simulink model "FieldOrientedControl"  (R2022b)
settings: configuration reference "FieldOrientedControl_ConfigSet" (kept outside this file)
PreLoadFcn:
  | run_start;
undefined symbols (not defined in the file or in its folder): DiscIntNeverNeededParam, dq_decouping_ena, dq_voltage_ratio, duty_sat_lower, duty_sat_upper, I_s_max, KI_c, Kp_c, L_d, L_q, p, Psi_p, svpwm_ena, task_time_mtrctrl
libraries: simulink x4
settings Model: DataDictionary=FieldOrientedControl.sldd  Creator=ext-turaim  LastModifiedBy=Musaab
settings ConfigSetRef: SourceName=FieldOrientedControl_ConfigSet

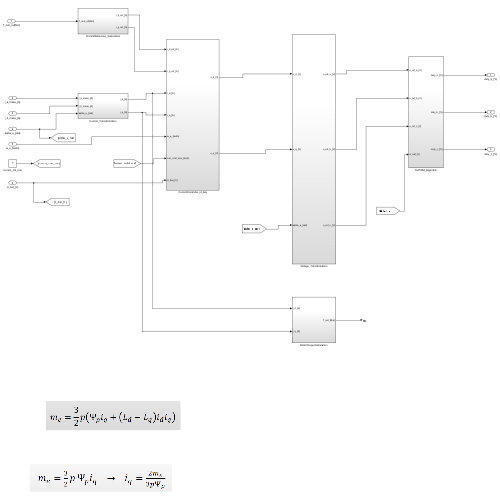
[thumbnail: Simulink's stored preview of the top-level diagram]
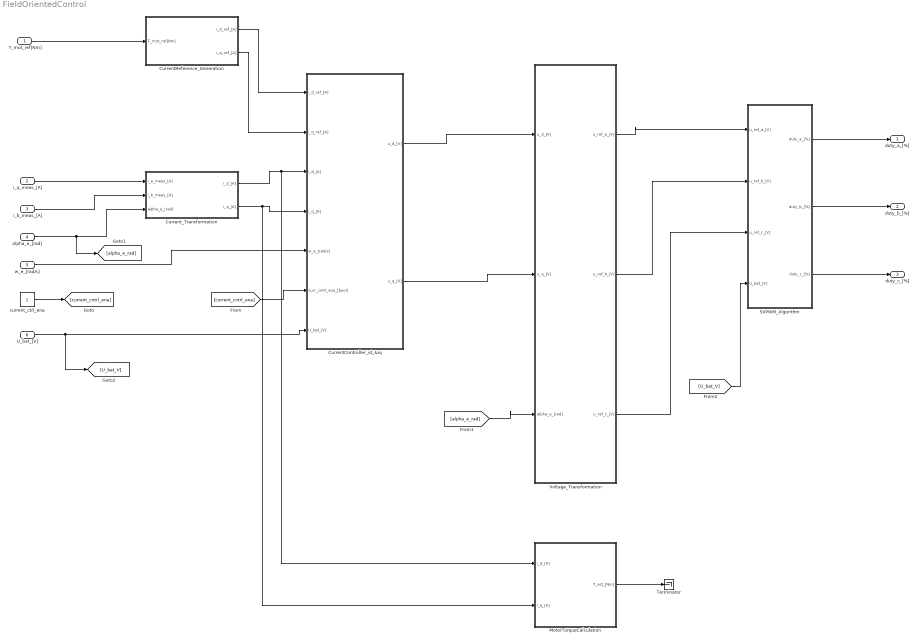
== system FieldOrientedControl ==
  T_mot_ref[Nm] : Inport  OutDataTypeStr=single  SampleTime=task_time_mtrctrl
  i_a_meas_[A] : Inport  Port=2  SampleTime=task_time_mtrctrl
  i_b_meas_[A] : Inport  Port=3  SampleTime=task_time_mtrctrl
  alpha_e_[rad] : Inport  Port=4  OutDataTypeStr=single  SampleTime=task_time_mtrctrl
  w_e_[rad/s] : Inport  Port=5  OutDataTypeStr=single  SampleTime=task_time_mtrctrl
  U_bat_[V] : Inport  Port=6  OutDataTypeStr=single  SampleTime=task_time_mtrctrl
  CurrentController_id_&iq : Subsystem
  CurrentReference_Generation : Subsystem
  Current_Transformation : Subsystem
  MotorTorqueCalculation : Subsystem
  SVPWM_Algorithm : Subsystem
  Terminator : Terminator
  Voltage_Transformation : Subsystem
  current_ctrl_ena : Constant  OutDataTypeStr=boolean  SampleTime=task_time_mtrctrl
  duty_a_[%] : Outport
  duty_b_[%] : Outport  Port=2
  duty_c_[%] : Outport  Port=3
  wires:
  i_a_meas_[A]/1 -> Current_Transformation/1(i_a_meas_[A])
  i_b_meas_[A]/1 -> Current_Transformation/2(i_b_meas_[A])
  alpha_e_[rad]/1 -> [alpha_e_rad], Current_Transformation/3(alpha_e_[rad])
  T_mot_ref[Nm]/1 -> CurrentReference_Generation/1(T_mot_ref[Nm])
  CurrentReference_Generation/1(i_d_ref_[A]) -> CurrentController_id_&iq/1(i_d_ref_[A])
  CurrentReference_Generation/2(i_q_ref_[A]) -> CurrentController_id_&iq/2(i_q_ref_[A])
  Current_Transformation/1(i_d_[A]) -> MotorTorqueCalculation/1(i_d_[A]), CurrentController_id_&iq/3(i_d_[A])
  Current_Transformation/2(i_q_[A]) -> MotorTorqueCalculation/2(i_q_[A]), CurrentController_id_&iq/4(i_q_[A])
  current_ctrl_ena/1 -> [current_cntrl_ena]
  [current_cntrl_ena] -> CurrentController_id_&iq/6(curr_cntrl_ena_[bool])
  w_e_[rad/s]/1 -> CurrentController_id_&iq/5(w_e_[rad/s])
  U_bat_[V]/1 -> [U_bat_V], CurrentController_id_&iq/7(U_bat_[V])
  CurrentController_id_&iq/1(u_d_[V]) -> Voltage_Transformation/1(u_d_[V])
  CurrentController_id_&iq/2(u_q_[V]) -> Voltage_Transformation/2(u_q_[V])
  [alpha_e_rad] -> Voltage_Transformation/3(alpha_e_[rad])
  Voltage_Transformation/1(u_ref_a_[V]) -> SVPWM_Algorithm/1(u_ref_a_[V])
  Voltage_Transformation/2(u_ref_b_[V]) -> SVPWM_Algorithm/2(u_ref_b_[V])
  Voltage_Transformation/3(u_ref_c_[V]) -> SVPWM_Algorithm/3(u_ref_c_[V])
  [U_bat_V] -> SVPWM_Algorithm/4(U_bat_[V])
  SVPWM_Algorithm/1(duty_a_[%]) -> duty_a_[%]/1
  SVPWM_Algorithm/2(duty_b_[%]) -> duty_b_[%]/1
  SVPWM_Algorithm/3(duty_c_[%]) -> duty_c_[%]/1
  MotorTorqueCalculation/1(T_act_[Nm]) -> Terminator/1

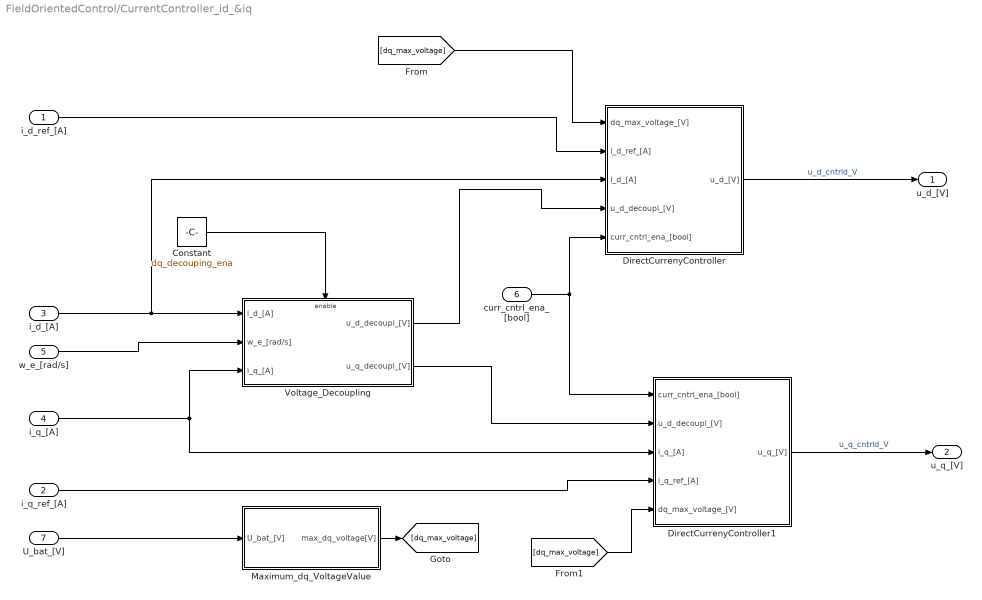
== system FieldOrientedControl/CurrentController_id_&iq ==
  i_d_ref_[A] : Inport
  i_q_ref_[A] : Inport  Port=2
  i_d_[A] : Inport  Port=3
  i_q_[A] : Inport  Port=4
  w_e_[rad/s] : Inport  Port=5
  curr_cntrl_ena_[bool] : Inport  Port=6
  U_bat_[V] : Inport  Port=7
  Constant : Constant  Value=dq_decouping_ena
  DirectCurrenyController : Subsystem
  DirectCurrenyController1 : Subsystem
  Maximum_dq_VoltageValue : Subsystem
  Voltage_Decoupling : Subsystem
  u_d_[V] : Outport
  u_q_[V] : Outport  Port=2
  wires:
  w_e_[rad/s]/1 -> Voltage_Decoupling/2(w_e_[rad/s])
  i_d_[A]/1 -> Voltage_Decoupling/1(i_d_[A]), DirectCurrenyController/3(i_d_[A])
  i_q_[A]/1 -> Voltage_Decoupling/3(i_q_[A]), DirectCurrenyController1/3(i_q_[A])
  i_d_ref_[A]/1 -> DirectCurrenyController/2(i_d_ref_[A])
  Voltage_Decoupling/1(u_d_decoupl_[V]) -> DirectCurrenyController/4(u_d_decoupl_[V])
  curr_cntrl_ena_[bool]/1 -> DirectCurrenyController1/1(curr_cntrl_ena_[bool]), DirectCurrenyController/5(curr_cntrl_ena_[bool])
  U_bat_[V]/1 -> Maximum_dq_VoltageValue/1(U_bat_[V])
  Maximum_dq_VoltageValue/1(max_dq_voltage[V]) -> [dq_max_voltage]
  [dq_max_voltage] -> DirectCurrenyController/1(dq_max_voltage_[V])
  DirectCurrenyController/1(u_d_[V]) -> u_d_[V]/1  "u_d_cntrld_V"
  [dq_max_voltage] -> DirectCurrenyController1/5(dq_max_voltage_[V])
  Voltage_Decoupling/2(u_q_decoupl_[V]) -> DirectCurrenyController1/2(u_d_decoupl_[V])
  i_q_ref_[A]/1 -> DirectCurrenyController1/4(i_q_ref_[A])
  DirectCurrenyController1/1(u_q_[V]) -> u_q_[V]/1  "u_q_cntrld_V"
  Constant/1 -> Voltage_Decoupling/Enable

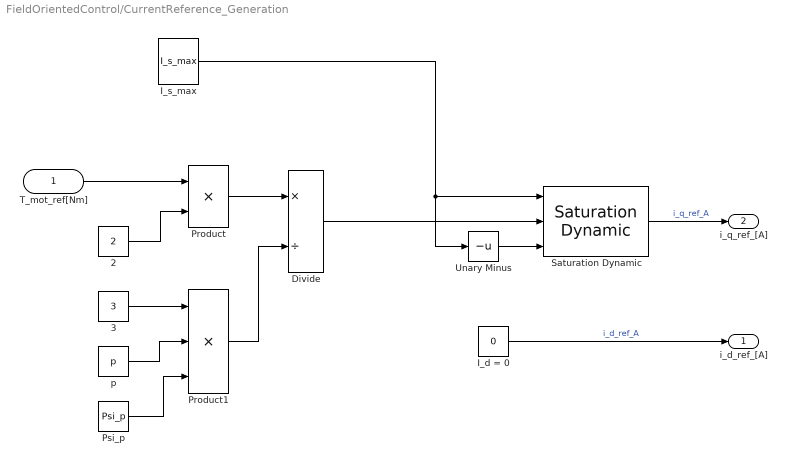
== system FieldOrientedControl/CurrentReference_Generation ==
  T_mot_ref[Nm] : Inport
  2 : Constant  Value=2  OutDataTypeStr=single
  3 : Constant  Value=3  OutDataTypeStr=single
  Divide : Product  Inputs=*/
  I_d = 0 : Constant  Value=0  OutDataTypeStr=single
  I_s_max : Constant  Value=I_s_max
  Product : Product
  Product1 : Product  Inputs=3
  Psi_p : Constant  Value=Psi_p  OutDataTypeStr=single
  Saturation Dynamic : simulink/Discontinuities/Saturation Dynamic  OutMin=[]  OutMax=[]  OutDataTypeStr=Inherit: Same as second input  OutDataType=fixdt(1, 16)  OutScaling=2^-10  DoSatur=off
  Unary Minus : UnaryMinus
  p : Constant  Value=p  OutDataTypeStr=single
  i_d_ref_[A] : Outport
  i_q_ref_[A] : Outport  Port=2
  wires:
  T_mot_ref[Nm]/1 -> Product/1
  2/1 -> Product/2
  3/1 -> Product1/1
  p/1 -> Product1/2
  Psi_p/1 -> Product1/3
  Product/1 -> Divide/1
  Product1/1 -> Divide/2
  I_s_max/1 -> Unary Minus/1, Saturation Dynamic/1
  Divide/1 -> Saturation Dynamic/2
  Saturation Dynamic/1 -> i_q_ref_[A]/1  "i_q_ref_A"
  Unary Minus/1 -> Saturation Dynamic/3
  I_d = 0/1 -> i_d_ref_[A]/1  "i_d_ref_A"

== system FieldOrientedControl/Current_Transformation ==
  i_a_meas_[A] : Inport
  i_b_meas_[A] : Inport  Port=2
  alpha_e_[rad] : Inport  Port=3
  Clark_Transformation : Subsystem
  Park_Transformation : Subsystem
  i_d_[A] : Outport
  i_q_[A] : Outport  Port=2
  wires:
  i_a_meas_[A]/1 -> Clark_Transformation/1(i_a_meas_[A])
  i_b_meas_[A]/1 -> Clark_Transformation/2(i_b_meas_[A])
  Clark_Transformation/1(i_x_[A]) -> Park_Transformation/1(i_x_[A])  "i_x_meas_A"
  Clark_Transformation/2(i_y_[A]) -> Park_Transformation/2(i_y_[A])  "i_y_meas_A"
  alpha_e_[rad]/1 -> Park_Transformation/3(alpha_e_[rad])
  Park_Transformation/1(i_d_[A]) -> i_d_[A]/1  "i_d_meas_A"
  Park_Transformation/2(i_q_[A]) -> i_q_[A]/1  "i_q_meas_A"

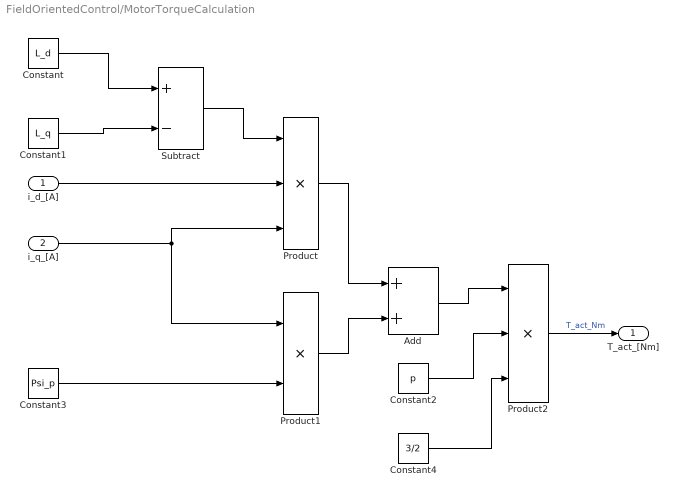
== system FieldOrientedControl/MotorTorqueCalculation ==
  i_d_[A] : Inport
  i_q_[A] : Inport  Port=2
  Add : Sum
  Constant : Constant  Value=L_d
  Constant1 : Constant  Value=L_q
  Constant2 : Constant  Value=p
  Constant3 : Constant  Value=Psi_p
  Constant4 : Constant  Value=3/2
  Product : Product  Inputs=3
  Product1 : Product
  Product2 : Product  Inputs=3
  Subtract : Sum  Inputs=+-
  T_act_[Nm] : Outport
  wires:
  Constant/1 -> Subtract/1
  Constant1/1 -> Subtract/2
  Subtract/1 -> Product/1
  i_d_[A]/1 -> Product/2
  i_q_[A]/1 -> Product1/1, Product/3
  Constant3/1 -> Product1/2
  Product/1 -> Add/1
  Product1/1 -> Add/2
  Add/1 -> Product2/1
  Constant2/1 -> Product2/2
  Constant4/1 -> Product2/3
  Product2/1 -> T_act_[Nm]/1  "T_act_Nm"

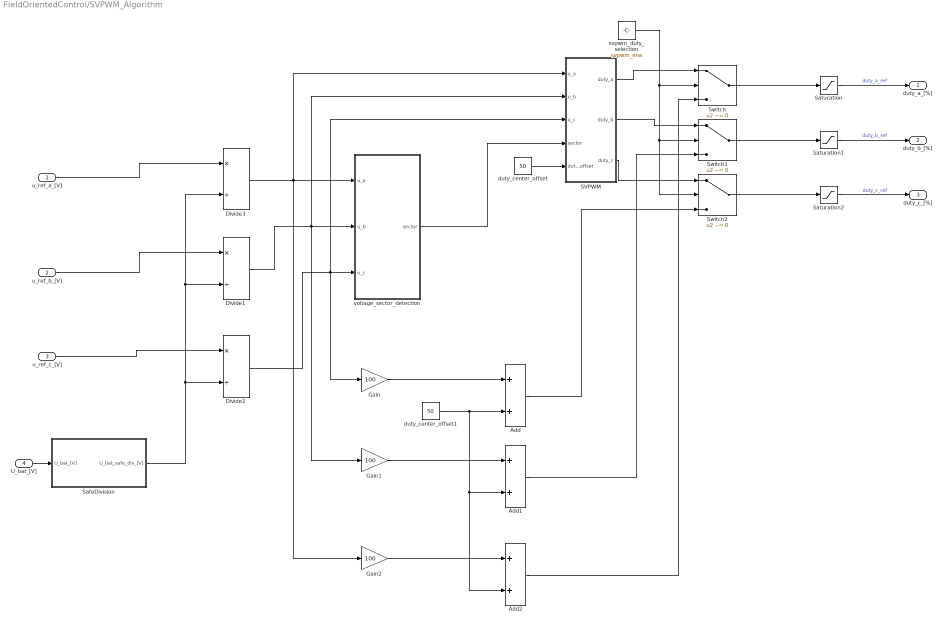
== system FieldOrientedControl/SVPWM_Algorithm ==
  u_ref_a_[V] : Inport
  u_ref_b_[V] : Inport  Port=2
  u_ref_c_[V] : Inport  Port=3
  U_bat_[V] : Inport  Port=4
  Add : Sum
  Add1 : Sum
  Add2 : Sum
  Divide1 : Product  Inputs=*/
  Divide2 : Product  Inputs=*/
  Divide3 : Product  Inputs=*/
  Gain : Gain  Gain=100
  Gain1 : Gain  Gain=100
  Gain2 : Gain  Gain=100
  SVPWM : Stateflow chart  TreatAsAtomicUnit=on
  SafeDivision : Subsystem
  Saturation : Saturate  UpperLimit=duty_sat_upper  LowerLimit=duty_sat_lower
  Saturation1 : Saturate  UpperLimit=duty_sat_upper  LowerLimit=duty_sat_lower
  Saturation2 : Saturate  UpperLimit=duty_sat_upper  LowerLimit=duty_sat_lower
  Switch : Switch  Criteria=u2 ~= 0  SaturateOnIntegerOverflow=off  InputSameDT=off
  Switch1 : Switch  Criteria=u2 ~= 0  SaturateOnIntegerOverflow=off  InputSameDT=off
  Switch2 : Switch  Criteria=u2 ~= 0  SaturateOnIntegerOverflow=off  InputSameDT=off
  duty_center_offset : Constant  Value=50  OutDataTypeStr=single
  duty_center_offset1 : Constant  Value=50  OutDataTypeStr=single
  svpwm_duty_selection : Constant  Value=svpwm_ena  OutDataTypeStr=single
  voltage_sector_detection : Stateflow chart  TreatAsAtomicUnit=on
  duty_a_[%] : Outport  OutDataTypeStr=single
  duty_b_[%] : Outport  Port=2  OutDataTypeStr=single
  duty_c_[%] : Outport  Port=3  OutDataTypeStr=single
  wires:
  U_bat_[V]/1 -> SafeDivision/1(U_bat_[V])
  u_ref_a_[V]/1 -> Divide3/1
  u_ref_b_[V]/1 -> Divide1/1
  u_ref_c_[V]/1 -> Divide2/1
  SafeDivision/1(U_bat_safe_div_[V]) -> Divide2/2, Divide1/2, Divide3/2
  Divide3/1 -> Gain2/1, voltage_sector_detection/1(u_a), SVPWM/1(u_a)
  Divide1/1 -> Gain1/1, voltage_sector_detection/2(u_b), SVPWM/2(u_b)
  Divide2/1 -> Gain/1, voltage_sector_detection/3(u_c), SVPWM/3(u_c)
  voltage_sector_detection/1(sector) -> SVPWM/4(sector)
  duty_center_offset/1 -> SVPWM/5(duty_offset)
  Gain/1 -> Add/1
  duty_center_offset1/1 -> Add2/2, Add1/2, Add/2
  Gain1/1 -> Add1/1
  Gain2/1 -> Add2/1
  SVPWM/1(duty_a) -> Switch/1
  SVPWM/2(duty_b) -> Switch1/1
  SVPWM/3(duty_c) -> Switch2/1
  Add2/1 -> Switch/3
  Add1/1 -> Switch1/3
  Add/1 -> Switch2/3
  svpwm_duty_selection/1 -> Switch1/2, Switch2/2, Switch/2
  Switch/1 -> Saturation/1
  Switch2/1 -> Saturation2/1
  Switch1/1 -> Saturation1/1
  Saturation2/1 -> duty_c_[%]/1  "duty_c_ref"
  Saturation1/1 -> duty_b_[%]/1  "duty_b_ref"
  Saturation/1 -> duty_a_[%]/1  "duty_a_ref"

== system FieldOrientedControl/Voltage_Transformation ==
  u_d_[V] : Inport
  u_q_[V] : Inport  Port=2
  alpha_e_[rad] : Inport  Port=3
  Inverse_Clarke_Transform : Subsystem
  Inverse_Park_Transform : Subsystem
  u_ref_a_[V] : Outport
  u_ref_b_[V] : Outport  Port=2
  u_ref_c_[V] : Outport  Port=3
  wires:
  u_d_[V]/1 -> Inverse_Park_Transform/1(u_d_[V])
  u_q_[V]/1 -> Inverse_Park_Transform/2(u_q_[V])
  alpha_e_[rad]/1 -> Inverse_Park_Transform/3(alpha_e_[rad])
  Inverse_Park_Transform/1(u_x_[V]) -> Inverse_Clarke_Transform/1(u_x_[V])  "u_x_V"
  Inverse_Park_Transform/2(u_y_[V]) -> Inverse_Clarke_Transform/2(u_y_[V])  "u_y_V"
  Inverse_Clarke_Transform/1(u_ref_a_[V]) -> u_ref_a_[V]/1  "u_ref_a_V"
  Inverse_Clarke_Transform/2(u_ref_b_[V]) -> u_ref_b_[V]/1  "u_ref_b_V"
  Inverse_Clarke_Transform/3(u_ref_c_[V]) -> u_ref_c_[V]/1  "u_ref_c_V"

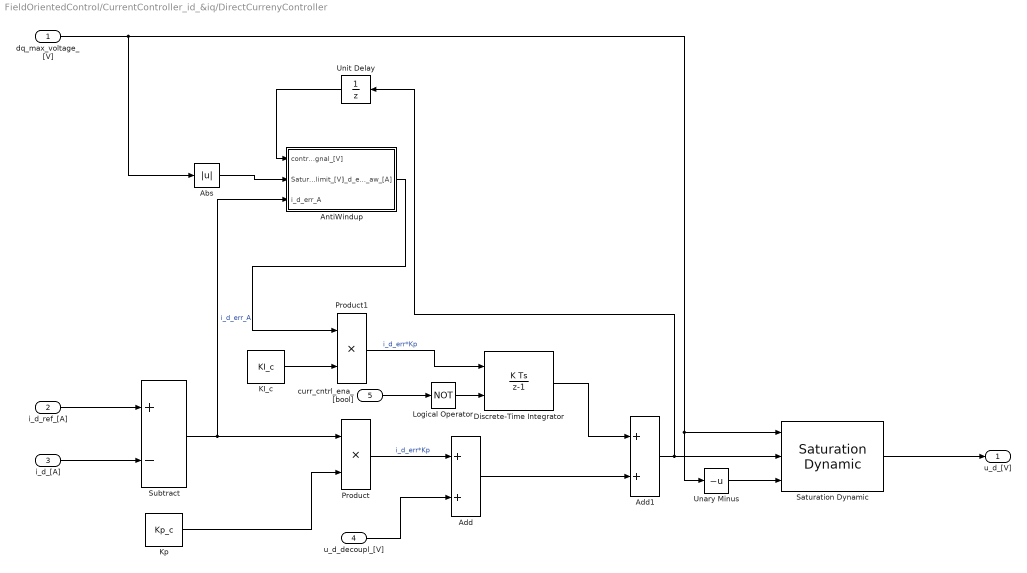
== system FieldOrientedControl/CurrentController_id_&iq/DirectCurrenyController ==
  dq_max_voltage_[V] : Inport
  i_d_ref_[A] : Inport  Port=2
  i_d_[A] : Inport  Port=3
  u_d_decoupl_[V] : Inport  Port=4
  curr_cntrl_ena_[bool] : Inport  Port=5
  Abs : Abs  SaturateOnIntegerOverflow=off
  Add : Sum
  Add1 : Sum
  AntiWindup : Subsystem
  Discrete-Time Integrator : DiscreteIntegrator  ExternalReset=level  SampleTime=-1  ICPrevOutput=DiscIntNeverNeededParam  ICPrevScaledInput=DiscIntNeverNeededParam
  KI_c : Constant  Value=KI_c
  Kp : Constant  Value=Kp_c
  Logical Operator : Logic  Operator=NOT  AllPortsSameDT=off  OutDataTypeStr=boolean
  Product : Product
  Product1 : Product
  Saturation Dynamic : simulink/Discontinuities/Saturation Dynamic  OutMin=[]  OutMax=[]  OutDataTypeStr=Inherit: Same as second input  OutDataType=fixdt(1, 16)  OutScaling=2^-10  DoSatur=off
  Subtract : Sum  Inputs=+-
  Unary Minus : UnaryMinus
  Unit Delay : UnitDelay  SampleTime=-1  HasFrameUpgradeWarning=on
  u_d_[V] : Outport
  wires:
  i_d_ref_[A]/1 -> Subtract/1
  i_d_[A]/1 -> Subtract/2
  Kp/1 -> Product/2
  Subtract/1 -> Product/1, AntiWindup/3(i_d_err_A)  "i_d_err_A"
  Product/1 -> Add/1  "i_d_err*Kp"
  u_d_decoupl_[V]/1 -> Add/2
  KI_c/1 -> Product1/2
  Product1/1 -> Discrete-Time Integrator/1  "i_d_err*Kp"
  Logical Operator/1 -> Discrete-Time Integrator/2
  curr_cntrl_ena_[bool]/1 -> Logical Operator/1
  Add/1 -> Add1/2
  Discrete-Time Integrator/1 -> Add1/1
  Add1/1 -> Unit Delay/1, Saturation Dynamic/2
  dq_max_voltage_[V]/1 -> Abs/1, Unary Minus/1, Saturation Dynamic/1
  Unary Minus/1 -> Saturation Dynamic/3
  Saturation Dynamic/1 -> u_d_[V]/1
  Unit Delay/1 -> AntiWindup/1(control_signal_[V])
  Abs/1 -> AntiWindup/2(Saturation_limit_[V])
  AntiWindup/1(i_d_err_aw_[A]) -> Product1/1

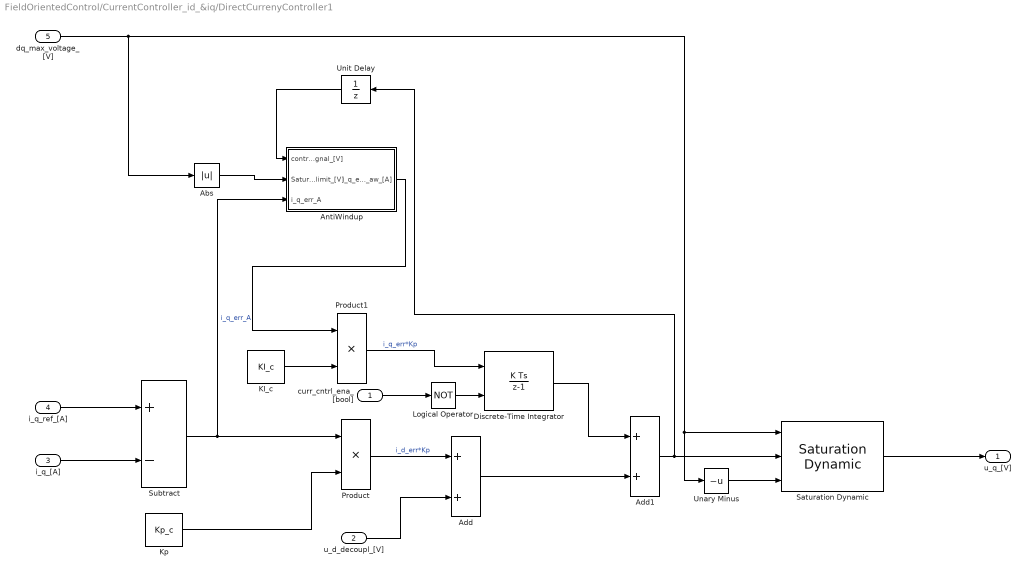
== system FieldOrientedControl/CurrentController_id_&iq/DirectCurrenyController1 ==
  curr_cntrl_ena_[bool] : Inport
  u_d_decoupl_[V] : Inport  Port=2
  i_q_[A] : Inport  Port=3
  i_q_ref_[A] : Inport  Port=4
  dq_max_voltage_[V] : Inport  Port=5
  Abs : Abs  SaturateOnIntegerOverflow=off
  Add : Sum
  Add1 : Sum
  AntiWindup : Subsystem
  Discrete-Time Integrator : DiscreteIntegrator  ExternalReset=level  SampleTime=-1  ICPrevOutput=DiscIntNeverNeededParam  ICPrevScaledInput=DiscIntNeverNeededParam
  KI_c : Constant  Value=KI_c
  Kp : Constant  Value=Kp_c
  Logical Operator : Logic  Operator=NOT  AllPortsSameDT=off  OutDataTypeStr=boolean
  Product : Product
  Product1 : Product
  Saturation Dynamic : simulink/Discontinuities/Saturation Dynamic  OutMin=[]  OutMax=[]  OutDataTypeStr=Inherit: Same as second input  OutDataType=fixdt(1, 16)  OutScaling=2^-10  DoSatur=off
  Subtract : Sum  Inputs=+-
  Unary Minus : UnaryMinus
  Unit Delay : UnitDelay  SampleTime=-1  HasFrameUpgradeWarning=on
  u_q_[V] : Outport
  wires:
  AntiWindup/1(i_q_err_aw_[A]) -> Product1/1
  Abs/1 -> AntiWindup/2(Saturation_limit_[V])
  Unit Delay/1 -> AntiWindup/1(control_signal_[V])
  Saturation Dynamic/1 -> u_q_[V]/1
  Unary Minus/1 -> Saturation Dynamic/3
  dq_max_voltage_[V]/1 -> Saturation Dynamic/1, Unary Minus/1, Abs/1
  Add1/1 -> Saturation Dynamic/2, Unit Delay/1
  Discrete-Time Integrator/1 -> Add1/1
  Add/1 -> Add1/2
  curr_cntrl_ena_[bool]/1 -> Logical Operator/1
  Logical Operator/1 -> Discrete-Time Integrator/2
  Product1/1 -> Discrete-Time Integrator/1  "i_q_err*Kp"
  KI_c/1 -> Product1/2
  u_d_decoupl_[V]/1 -> Add/2
  Product/1 -> Add/1  "i_d_err*Kp"
  Subtract/1 -> AntiWindup/3(i_q_err_A), Product/1  "i_q_err_A"
  Kp/1 -> Product/2
  i_q_[A]/1 -> Subtract/2
  i_q_ref_[A]/1 -> Subtract/1

== system FieldOrientedControl/CurrentController_id_&iq/Maximum_dq_VoltageValue ==
  U_bat_[V] : Inport
  1/sqrt(3) : Constant  Value=dq_voltage_ratio
  Product : Product
  max_dq_voltage[V] : Outport
  wires:
  U_bat_[V]/1 -> Product/1
  Product/1 -> max_dq_voltage[V]/1  "dq_max_voltage_V"
  1/sqrt(3)/1 -> Product/2

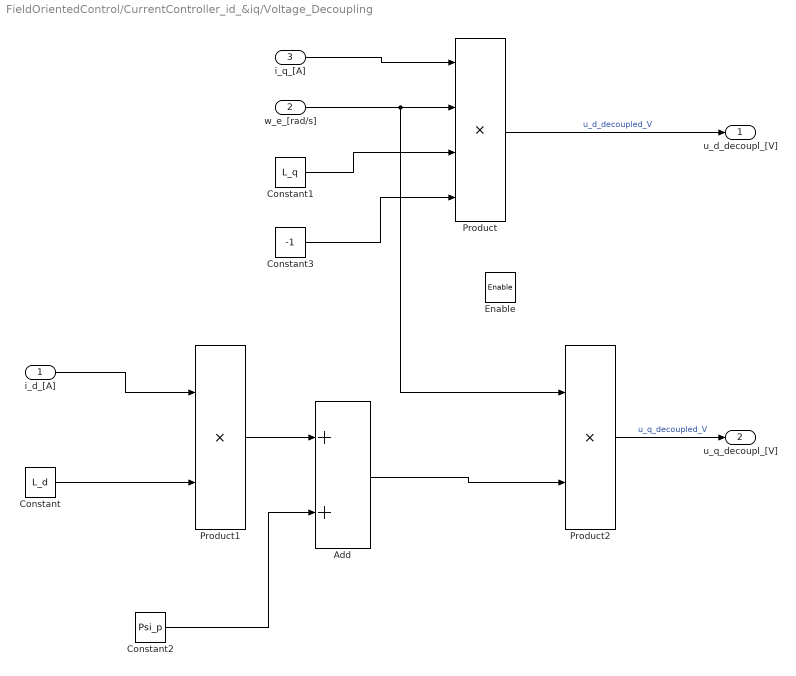
== system FieldOrientedControl/CurrentController_id_&iq/Voltage_Decoupling ==
  i_d_[A] : Inport
  w_e_[rad/s] : Inport  Port=2
  i_q_[A] : Inport  Port=3
  Enable : EnablePort
  Add : Sum
  Constant : Constant  Value=L_d
  Constant1 : Constant  Value=L_q
  Constant2 : Constant  Value=Psi_p
  Constant3 : Constant  Value=-1  OutDataTypeStr=single
  Product : Product  Inputs=4
  Product1 : Product
  Product2 : Product
  u_d_decoupl_[V] : Outport
  u_q_decoupl_[V] : Outport  Port=2
  wires:
  i_q_[A]/1 -> Product/1
  w_e_[rad/s]/1 -> Product2/1, Product/2
  Constant1/1 -> Product/3
  Constant3/1 -> Product/4
  Product/1 -> u_d_decoupl_[V]/1  "u_d_decoupled_V"
  i_d_[A]/1 -> Product1/1
  Constant/1 -> Product1/2
  Product1/1 -> Add/1
  Constant2/1 -> Add/2
  Add/1 -> Product2/2
  Product2/1 -> u_q_decoupl_[V]/1  "u_q_decoupled_V"

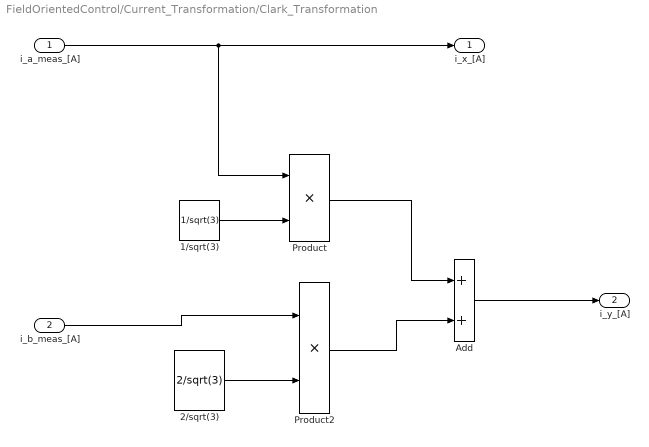
== system FieldOrientedControl/Current_Transformation/Clark_Transformation ==
  i_a_meas_[A] : Inport
  i_b_meas_[A] : Inport  Port=2
  1/sqrt(3) : Constant  Value=1/sqrt(3)  OutDataTypeStr=single
  2/sqrt(3) : Constant  Value=2/sqrt(3)  OutDataTypeStr=single
  Add : Sum
  Product : Product
  Product2 : Product
  i_x_[A] : Outport
  i_y_[A] : Outport  Port=2
  wires:
  i_a_meas_[A]/1 -> Product/1, i_x_[A]/1
  1/sqrt(3)/1 -> Product/2
  i_b_meas_[A]/1 -> Product2/1
  2/sqrt(3)/1 -> Product2/2
  Product/1 -> Add/1
  Product2/1 -> Add/2
  Add/1 -> i_y_[A]/1

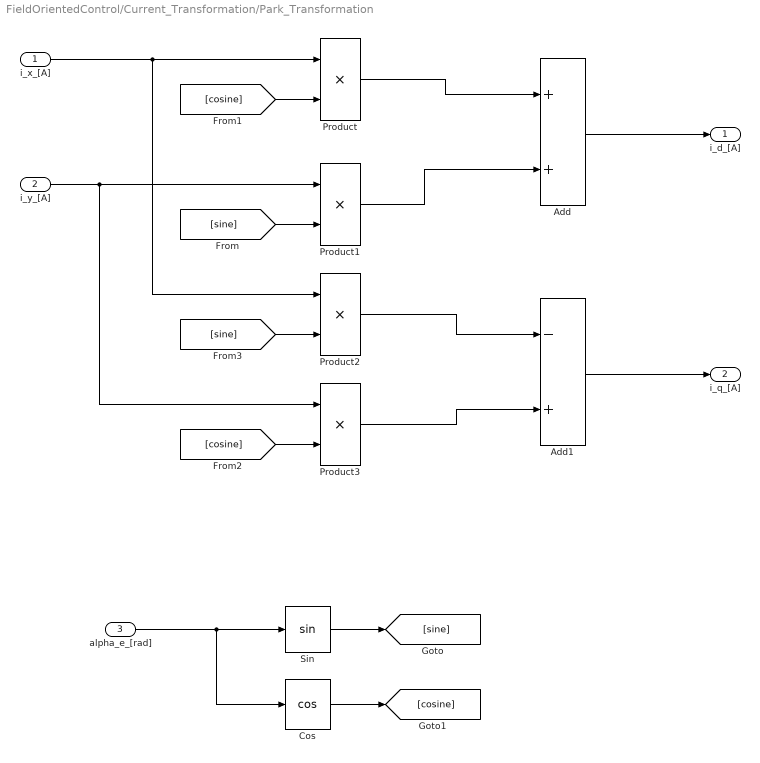
== system FieldOrientedControl/Current_Transformation/Park_Transformation ==
  i_x_[A] : Inport
  i_y_[A] : Inport  Port=2
  alpha_e_[rad] : Inport  Port=3
  Add : Sum
  Add1 : Sum  Inputs=-+
  Cos : Trigonometry  Operator=cos
  Product{,1..3} (4 alike) : Product
  Sin : Trigonometry
  i_d_[A] : Outport
  i_q_[A] : Outport  Port=2
  wires:
  alpha_e_[rad]/1 -> Cos/1, Sin/1
  Sin/1 -> [sine]
  Cos/1 -> [cosine]
  i_x_[A]/1 -> Product2/1, Product/1
  [cosine] -> Product/2
  i_y_[A]/1 -> Product3/1, Product1/1
  [cosine] -> Product3/2
  [sine] -> Product2/2
  [sine] -> Product1/2
  Product/1 -> Add/1
  Product1/1 -> Add/2
  Add/1 -> i_d_[A]/1
  Product2/1 -> Add1/1
  Product3/1 -> Add1/2
  Add1/1 -> i_q_[A]/1

== system FieldOrientedControl/SVPWM_Algorithm/SafeDivision ==
  U_bat_[V] : Inport
  Compare To Constant : simulink/Logic and Bit Operations/Compare To Constant  relop===  const=0  OutDataTypeStr=boolean
  Constant : Constant  Value=1e-6
  Switch : Switch  Criteria=u2 ~= 0  SaturateOnIntegerOverflow=off  InputSameDT=off
  U_bat_safe_div_[V] : Outport
  wires:
  Compare To Constant/1 -> Switch/2
  U_bat_[V]/1 -> Switch/3, Compare To Constant/1
  Constant/1 -> Switch/1
  Switch/1 -> U_bat_safe_div_[V]/1

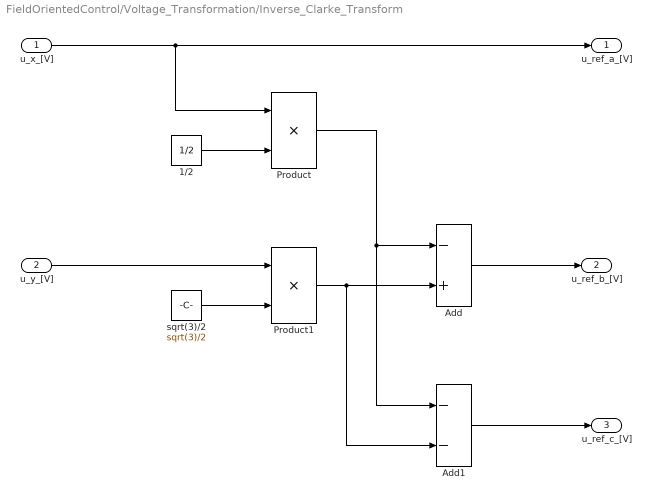
== system FieldOrientedControl/Voltage_Transformation/Inverse_Clarke_Transform ==
  u_x_[V] : Inport
  u_y_[V] : Inport  Port=2
  1/2 : Constant  Value=1/2  OutDataTypeStr=single
  Add : Sum  Inputs=-+
  Add1 : Sum  Inputs=--
  Product : Product
  Product1 : Product
  sqrt(3)/2 : Constant  Value=sqrt(3)/2  OutDataTypeStr=single
  u_ref_a_[V] : Outport
  u_ref_b_[V] : Outport  Port=2
  u_ref_c_[V] : Outport  Port=3
  wires:
  u_x_[V]/1 -> Product/1, u_ref_a_[V]/1
  1/2/1 -> Product/2
  sqrt(3)/2/1 -> Product1/2
  u_y_[V]/1 -> Product1/1
  Product1/1 -> Add1/2, Add/2
  Product/1 -> Add1/1, Add/1
  Add/1 -> u_ref_b_[V]/1
  Add1/1 -> u_ref_c_[V]/1

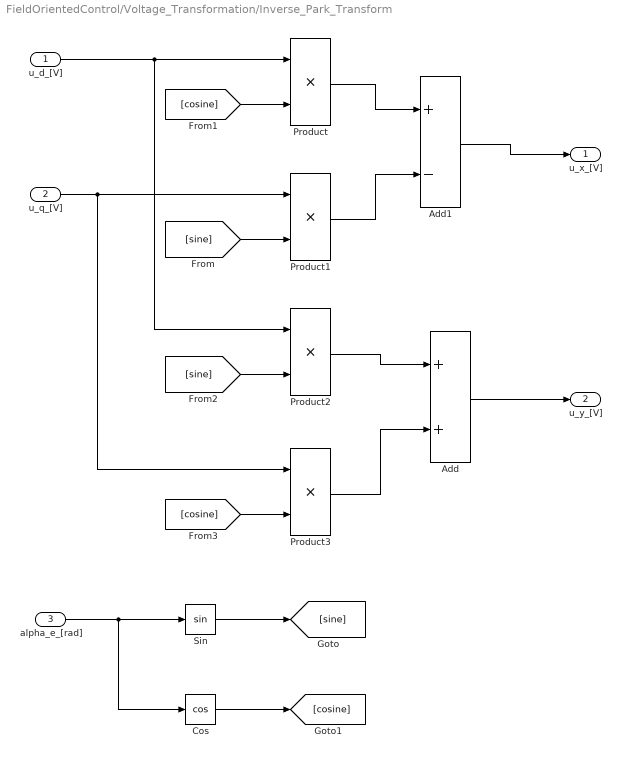
== system FieldOrientedControl/Voltage_Transformation/Inverse_Park_Transform ==
  u_d_[V] : Inport
  u_q_[V] : Inport  Port=2
  alpha_e_[rad] : Inport  Port=3
  Add : Sum
  Add1 : Sum  Inputs=+-
  Cos : Trigonometry  Operator=cos
  Product{,1..3} (4 alike) : Product
  Sin : Trigonometry
  u_x_[V] : Outport
  u_y_[V] : Outport  Port=2
  wires:
  alpha_e_[rad]/1 -> Cos/1, Sin/1
  Sin/1 -> [sine]
  Cos/1 -> [cosine]
  u_d_[V]/1 -> Product2/1, Product/1
  [sine] -> Product1/2
  [cosine] -> Product/2
  u_q_[V]/1 -> Product3/1, Product1/1
  [sine] -> Product2/2
  [cosine] -> Product3/2
  Product2/1 -> Add/1
  Product3/1 -> Add/2
  Add/1 -> u_y_[V]/1
  Product/1 -> Add1/1
  Product1/1 -> Add1/2
  Add1/1 -> u_x_[V]/1

== system FieldOrientedControl/CurrentController_id_&iq/DirectCurrenyController/AntiWindup ==
  control_signal_[V] : Inport
  Saturation_limit_[V] : Inport  Port=2
  i_d_err_A : Inport  Port=3
  Abs : Abs  SaturateOnIntegerOverflow=off
  Product : Product
  Relational Operator : RelationalOperator  Operator=<  OutDataTypeStr=boolean  RndMeth=Simplest  InputSameDT=off
  i_d_err_aw_[A] : Outport
  wires:
  control_signal_[V]/1 -> Abs/1
  Abs/1 -> Relational Operator/1
  Saturation_limit_[V]/1 -> Relational Operator/2
  Relational Operator/1 -> Product/1
  i_d_err_A/1 -> Product/2
  Product/1 -> i_d_err_aw_[A]/1

== system FieldOrientedControl/CurrentController_id_&iq/DirectCurrenyController1/AntiWindup ==
  control_signal_[V] : Inport
  Saturation_limit_[V] : Inport  Port=2
  i_q_err_A : Inport  Port=3
  Abs : Abs  SaturateOnIntegerOverflow=off
  Product : Product
  Relational Operator : RelationalOperator  Operator=<  OutDataTypeStr=boolean  RndMeth=Simplest  InputSameDT=off
  i_q_err_aw_[A] : Outport
  wires:
  Product/1 -> i_q_err_aw_[A]/1
  i_q_err_A/1 -> Product/2
  Relational Operator/1 -> Product/1
  Saturation_limit_[V]/1 -> Relational Operator/2
  Abs/1 -> Relational Operator/1
  control_signal_[V]/1 -> Abs/1

== stateflow chart FieldOrientedControl/SVPWM_Algorithm/SVPWM ==
  note: ?
  (default) -> (junction 15)
  (junction 15) -> (junction 17) [order 1] : [sector == 1 || sector == 4]{
      |
      | duty_a = duty_offset + duty_offset*(u_a - u_c);
      | duty_b = duty_offset + duty_offset*(2*u_b - u_a - u_c);
      | duty_c = duty_offset + duty_offset*(u_c - u_a);
      |
      | }
  (junction 15) -> (junction 19) [order 2]
  (junction 19) -> (junction 20) [order 1] : [sector == 2 || sector == 5]{
      |
      | duty_a = duty_offset + duty_offset*(2*u_a - u_b - u_c);
      | duty_b = duty_offset + duty_offset*(u_b - u_c);
      | duty_c = duty_offset + duty_offset*(u_c - u_b);
      |
      | }
  (junction 19) -> (junction 23) [order 2]
  (junction 23) -> (junction 24) : [sector == 3 || sector == 6]{
      |
      | duty_a = duty_offset + duty_offset*(u_a - u_b);
      | duty_b = duty_offset + duty_offset*(u_b - u_a);
      | duty_c = duty_offset + duty_offset*(2*u_c - u_a - u_b);
      |
      | }
  data: u_a input; u_b input; u_c input; sector input; duty_a output; duty_b output; duty_c output; duty_offset input

== stateflow chart FieldOrientedControl/SVPWM_Algorithm/voltage_sector_detection ==
  (default) -> (junction 4)
  (junction 4) -> (junction 20) [order 2]
  (junction 4) -> (junction 6) [order 1] : [u_a >= u_b]
  (junction 20) -> (junction 21)
  (junction 21) -> (junction 22) [order 1] : [u_a >= u_c]{sector = 2}
  (junction 6) -> (junction 7) [order 1] : [u_c >= u_a]{sector = 5}
  (junction 6) -> (junction 11) [order 2]
  (junction 21) -> (junction 26) [order 2]
  (junction 26) -> (junction 27) [order 1] : [u_b >= u_c]{sector = 3}
  (junction 26) -> (junction 31) [order 2]
  (junction 11) -> (junction 14) [order 1] : [u_c >= u_b]{sector = 6}
  (junction 11) -> (junction 16) [order 2]
  (junction 16) -> (junction 17) : {sector = 1}
  (junction 31) -> (junction 32) : {sector = 4}
  data: u_a input; u_b input; u_c input; sector output
